simulink model "test_on_intes_cross2018"  (R2018b)
settings: Solver=FixedStepAuto  StartTime=0.0  StopTime=20  FixedStep=0.001  RelTol=1e-3
libraries: simulink x1
settings Model: Creator=lenovo  LastModifiedBy=lenovo

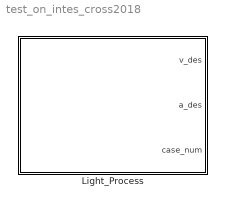
== system test_on_intes_cross2018 ==
  Light_Process : Subsystem

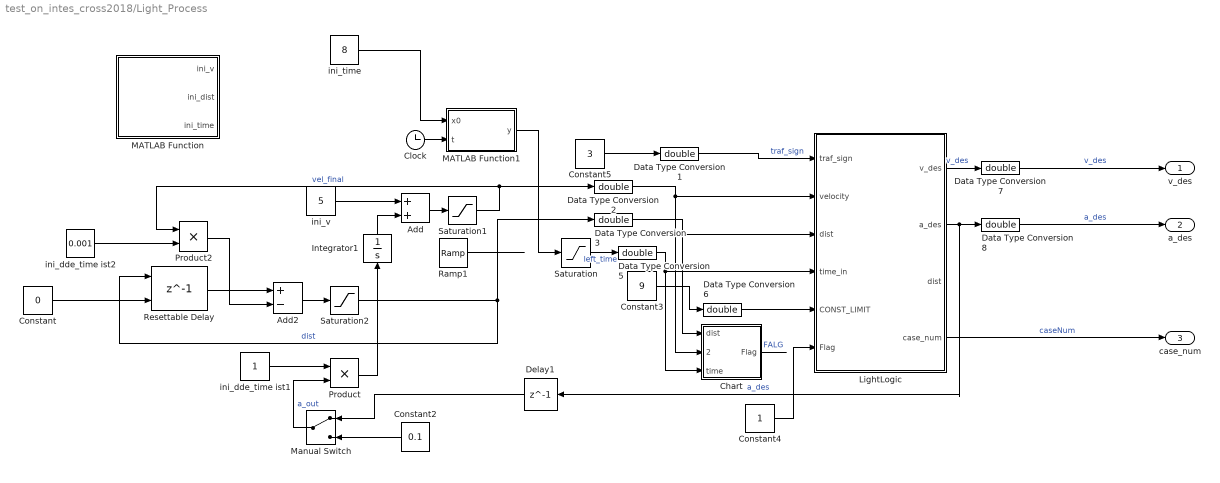
== system test_on_intes_cross2018/Light_Process ==
  Add : Sum
  Add2 : Sum  Inputs=+-
  Chart : Stateflow chart  TreatAsAtomicUnit=on
  Clock : Clock
  Constant : Constant  Value=0  OutDataTypeStr=single
  Constant2 : Constant  Value=0.1  OutDataTypeStr=single
  Constant3 : Constant  Value=9  OutDataTypeStr=single
  Constant4 : Constant  OutDataTypeStr=single
  Constant5 : Constant  Value=3  OutDataTypeStr=single
  Data Type Conversion{1..3,5..8} (7 alike) : DataTypeConversion  OutDataTypeStr=double
  Delay1 : Delay  DelayLength=1
  Integrator1 : Integrator
  LightLogic : MATLAB Function  TreatAsAtomicUnit=on
  MATLAB Function : MATLAB Function  TreatAsAtomicUnit=on
  MATLAB Function1 : MATLAB Function  TreatAsAtomicUnit=on
  Manual Switch : ManualSwitch
  Product : Product
  Product2 : Product
  Ramp1 : simulink/Sources/Ramp  slope=-1  start=0  InitialOutput=8
  Resettable Delay : Delay  DelayLength=1  InitialConditionSource=Input port
      settings: InputPortMap=u0,p4
  Saturation : Saturate  UpperLimit=40  LowerLimit=0
  Saturation1 : Saturate  UpperLimit=inf  LowerLimit=0
  Saturation2 : Saturate  UpperLimit=inf  LowerLimit=-10
  ini_dde_time ist1 : Constant  OutDataTypeStr=single
  ini_dde_time ist2 : Constant  Value=0.001  OutDataTypeStr=single
  ini_time : Constant  Value=8  OutDataTypeStr=single
  "ini_v " : Constant  Value=5  OutDataTypeStr=single
  v_des : Outport
  a_des : Outport  Port=2
  case_num : Outport  Port=3
  wires:
  Data Type Conversion7/1 -> v_des/1  "v_des"
  Data Type Conversion8/1 -> a_des/1  "a_des"
  "ini_v "/1 -> Add/1
  Data Type Conversion1/1 -> LightLogic/1(traf_sign)  "traf_sign"
  Data Type Conversion3/1 -> LightLogic/3("dist "), Chart/1(dist)
  Data Type Conversion5/1 -> LightLogic/4(time_in), Chart/3(time)
  Data Type Conversion6/1 -> LightLogic/5(CONST_LIMIT)
  LightLogic/1(v_des) -> Data Type Conversion7/1  "v_des"
  LightLogic/2(a_des) -> Delay1/1, Data Type Conversion8/1  "a_des"
  LightLogic/4(case_num) -> case_num/1  "caseNum"
  Chart/1(Flag) -> ?  "FALG"
  Constant5/1 -> Data Type Conversion1/1
  Ramp1/1 -> ?
  Constant3/1 -> Data Type Conversion6/1
  Add/1 -> Saturation1/1
  Saturation/1 -> Data Type Conversion5/1  "left_time"
  Add2/1 -> Saturation2/1
  Manual Switch/1 -> Product/2  "a_out"
  Constant2/1 -> Manual Switch/2
  Delay1/1 -> Manual Switch/1
  Integrator1/1 -> Add/2
  ini_dde_time ist1/1 -> Product/1
  Product/1 -> Integrator1/1
  Resettable Delay/1 -> Add2/1
  ini_dde_time ist2/1 -> Product2/2
  Product2/1 -> Add2/2
  Constant4/1 -> LightLogic/6(Flag)
  Data Type Conversion2/1 -> LightLogic/2(velocity), Chart/2(velocity)
  Saturation1/1 -> Product2/1, Data Type Conversion2/1  "vel_final"
  Saturation2/1 -> Resettable Delay/1, Data Type Conversion3/1  "dist"
  Constant/1 -> Resettable Delay/2
  Clock/1 -> MATLAB Function1/2(t)
  MATLAB Function1/1(y) -> Saturation/1
  ini_time/1 -> MATLAB Function1/1(x0)

== stateflow chart test_on_intes_cross2018/Light_Process/Chart ==
  state init
    en:
    Flag=0;
  state Off
    en:
    Flag=0;
  state On
    du:
    Flag=1;
  (default) -> init
  Off -> init : [time > 0 && dist > 0]
  init -> On : [(time > 0 && dist > 0 && dist / (velocity + 0.0001) <= 5)]
  On -> Off : [dist < -5 || time < 0]
  data: dist input; velocity input; Flag output; time input

== matlab function test_on_intes_cross2018/Light_Process/MATLAB Function ==
  data: ini_v output; ini_dist output; ini_time output
function [ini_v,ini_dist,ini_time]    = fcn

for ini_v = 5:20
    for ini_dist = 20:60
        for ini_time = 5:15
            
        end
    end
end
end

== matlab function test_on_intes_cross2018/Light_Process/MATLAB Function1 ==
  data: x0 input; y output; t input
function y = fcn(x0, t)

y = x0 - t ;

== matlab function test_on_intes_cross2018/Light_Process/LightLogic ==
  data: v_des output; a_des output; traf_sign input; velocity input; dist input; time_in input; CONST_LIMIT input; dist output; case_num output; Flag input
function [v_des,a_des,dist,case_num] = intesec_cross( traf_sign, velocity, dist, time_in,CONST_LIMIT,Flag)  
%% this is a function that provide desired velocity, and distance to traffic light;
    % input: trafic_sign with green = 0; red = 1; yellow = 2;
    %        velocity in unit of kph;
    %        dist, and time is distance(m) to cross, and traffic time left
    %        CONST_LIMIT is velocity limit at cross, which is a reference CONSTANT velocity from
    %        ACC module.
    %        v_des_pre preseve previous v_des for next step use.
    
    % output: desired velocity for ACC module, in unit of kph;
    %         dist is distance(m) to front cross;
   
    case_num = 0;
    time = time_in;
    green = 1;
    red = 3;
    yellow = 2;
%     if time == 2
%         a_des = 0;
%          v_des = 0;
%     end
    
    if (Flag == 0)
        v_des = velocity;
        a_des = 0.5;
        dist = dist;
        case_num = 0;
       
        
    else   %(Flag == 1)

        if dist < 0
            dist = 0; 
        end

        v = velocity;

        if traf_sign == green
            time = time + 3;
        elseif traf_sign == yellow
            traf_sign = green;
        end

        switch traf_sign
            case green
                T_ACC = (max(0,dist)+0.1) / (v + 0.0001);
                T_ACC_QUIT = (dist - 5) / (v + 0.0001);
                T = time;
                a = 2 * (dist - v * T) / (T^2 + 0.0001);
                v_temp = v + a * T;
                
                if dist == 200
                    v_des = 15;
                    a_des = 1;
                    case_num = 0;
                    return;
                end
                
                if T_ACC_QUIT > 8  && v < 2.5
                    v_des = 15;
                    a_des = 1;
                    case_num = 0;
                    return;
                end

                if T_ACC < T % green time is long enough
                    if v > CONST_LIMIT %
                        a0 =  (CONST_LIMIT^2 - v^2) / (2*dist + 0.001);
                        a0 = max(a0,-1);
                        vt = sqrt(max(0,v^2 + 2 * a0 * dist));
                        t0 = (vt - v) / (a0);
                        
                        if t0 <= T % decelerate to vt is OK
                            v_des = vt; % (v + t0 * a0);
                            a_des = a0;
                            case_num = 1;
                        else 
                            v_des = v + T * a0;
                            a_des = a0;
                            case_num = 2;
                        end
                    else % green 
                        v_des = CONST_LIMIT;
                        a_des = (CONST_LIMIT - v)/T;
                        case_num = 3;
                    end
                    
                else % ( T_ACC >= T)
                    if ((a >= 0) && (a < 1) && (v_temp <= CONST_LIMIT))
                        v_des = CONST_LIMIT;
                        a_des = a;
                        case_num = 4;
                    else
                        v_des  = 0;
                        a_des = -v^2 / (2 * dist); 
                        case_num = 5;
                    end
                end

            case red
                T_ACC_QUIT = (dist - 5) / (v + 0.0001);
                if T_ACC_QUIT > 10 && dist >= 5
                    v_des = 15;
                    a_des = 1;
                    case_num = 0;
                    return;
                end

                if (dist < 4) && (v < 1)
                    a_des = 0.25 * dist - 1;
                    v_des = 0;
                    case_num = 12;

                else
                    T = time;
                    T_ACC = dist / (v + 0.0001);
                    a = 2 * (dist - v * T) / (T+0.001)^2;
                    v_temp = v + a * T;

                    if T_ACC < T
                        a0 = -v^2 / (2 * dist);
                        t0 = -v / a0;
                        if t0 < time
                            v_des = 0;
                            a_des = max(-1, -v^2 / (2 * dist+ 0.01));
                            case_num = 7;
                        else
                            v_des = v_temp;
                            a_des = a;
                            case_num = 8;
                        end 

                    else % (T_ACC > T)
                        if (v_temp < CONST_LIMIT)
                            v_des = v_temp;
                            a_des = max(-1,a);
                            case_num = 9;
                        else
                            v_des = CONST_LIMIT;
                            a_des = (CONST_LIMIT - v) / T;
                            case_num = 10;
                        end

                    end
                end

               

            otherwise
                v_des = CONST_LIMIT;
                a_des = 0;
                case_num = 11;
        end
        
%     else
%         v_des = 100;
%         a_des = 100;
%         dist = 100;
%         case_num = 0;
%          
    end
end
